simulink model "Models"  (R2016b)
settings: Solver=FixedStepAuto  StartTime=0.0  StopTime=100  FixedStep=0.05  RelTol=1e-3
model workspace (MAT data in the model file):
  index = Simulink.Signal
  index.DataType = 'double'
  index.Dimensions = 1
  index.DimensionsMode = 'Fixed'
  index.Complexity = 'real'
  index.SampleTime = -1
  index.SamplingMode = 'auto'
  index.InitialValue = '1'
values from neighbouring files (symbols this model uses):
  dpitch = 7.203    [Parameters.m]
  droll = 0.1094    [Parameters.m]
  dx = 2.86    [Parameters.m]
  dyaw = 0.26285    [Parameters.m]
  dz = 0    [Parameters.m]
  F = Fe(1:2,1:3)    [ControllerLQR.m]    (also in robustModel.m = -info.KFI(1:2,1:3))
  Ix = 0.06541    [Parameters.m]
  Iy = 1.08921    [Parameters.m]
  Iz = 1.10675    [Parameters.m]    (also in robustModel.m = Iz-0.22)
  l1 = 0.05    [Parameters.m]
  l2 = 0.05    [Parameters.m]
  m = 13    [Parameters.m]    (also in robustModel.m = m-2.6)
  refXdot = 1    [ControllerLQR.m]    (also in robustModel.m)
  refYaw = 1    [ControllerLQR.m]    (also in robustModel.m)
  Tpitch = 131.8316    [Parameters.m]
  Troll = 6.9736    [Parameters.m]
undefined symbols (not defined in the file or in its folder): DiscIntNeverNeededParam, F1, F2, Fi
settings Model: Creator=USUARIO  LastModifiedBy=aleja
settings DataIOCC: Refine=100

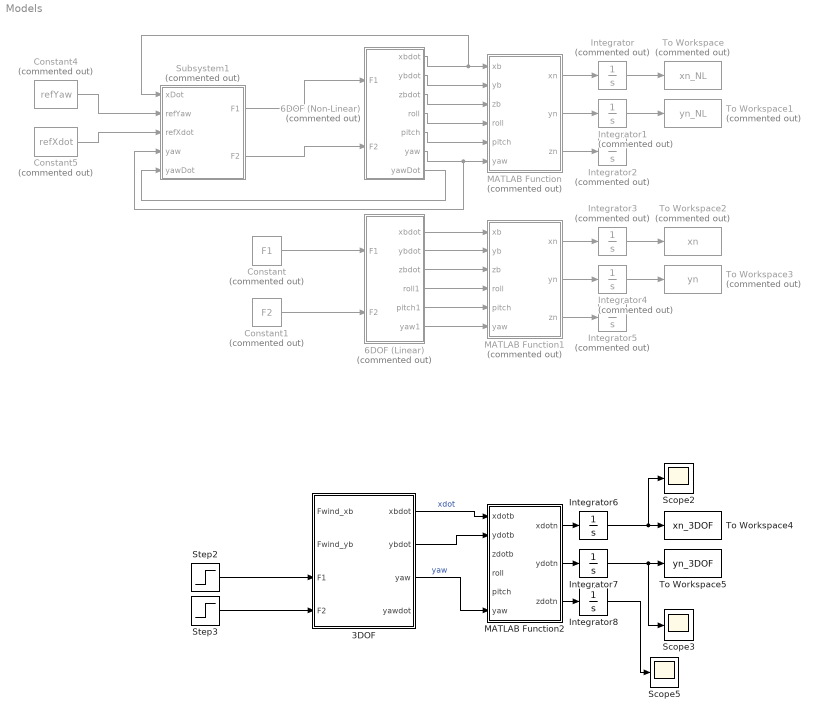
== system Models ==
  3DOF : Subsystem
  6DOF (Linear) : Subsystem  Commented=on
  6DOF (Non-Linear) : Subsystem  Commented=on
  Constant : Constant  Commented=on  Value=F1
  Constant1 : Constant  Commented=on  Value=F2
  Constant4 : Constant  Commented=on  Value=refYaw
  Constant5 : Constant  Commented=on  Value=refXdot
  Integrator{,1..5} (6 alike) : Integrator  Commented=on
  Integrator6 : Integrator
  Integrator7 : Integrator
  Integrator8 : Integrator
  MATLAB Function : MATLAB Function  Commented=on  TreatAsAtomicUnit=on
  MATLAB Function1 : MATLAB Function  Commented=on  TreatAsAtomicUnit=on
  MATLAB Function2 : MATLAB Function  TreatAsAtomicUnit=on
  Scope2 : Scope
  Scope3 : Scope
  Scope5 : Scope
  Step2 : Step  Time=10  After=14  SampleTime=0
  Step3 : Step  Time=10  After=14  SampleTime=0
  Subsystem1 : Subsystem  Commented=on
  To Workspace : ToWorkspace  Commented=on  VariableName=xn_NL  SaveFormat=Timeseries  SampleTime=-1
  To Workspace1 : ToWorkspace  Commented=on  VariableName=yn_NL  SaveFormat=Timeseries  SampleTime=-1
  To Workspace2 : ToWorkspace  Commented=on  VariableName=xn  SaveFormat=Timeseries  SampleTime=-1
  To Workspace3 : ToWorkspace  Commented=on  VariableName=yn  SaveFormat=Timeseries  SampleTime=-1
  To Workspace4 : ToWorkspace  VariableName=xn_3DOF  SaveFormat=Timeseries  SampleTime=-1
  To Workspace5 : ToWorkspace  VariableName=yn_3DOF  SaveFormat=Timeseries  SampleTime=-1
  wires:
  Constant/1 -> 6DOF (Linear)/1(F1)
  Constant1/1 -> 6DOF (Linear)/2(F2)
  MATLAB Function/1(xn) -> Integrator/1
  MATLAB Function/2(yn) -> Integrator1/1
  6DOF (Non-Linear)/6(yaw) -> Subsystem1/4(yaw), MATLAB Function/6(yaw)
  6DOF (Non-Linear)/5(pitch) -> MATLAB Function/5(pitch)
  6DOF (Non-Linear)/4(roll) -> MATLAB Function/4(roll)
  6DOF (Non-Linear)/3(zbdot) -> MATLAB Function/3(zb)
  6DOF (Non-Linear)/2(ybdot) -> MATLAB Function/2(yb)
  3DOF/1(xbdot) -> MATLAB Function2/1(xdotb)  "xdot"
  3DOF/2(ybdot) -> MATLAB Function2/2(ydotb)
  3DOF/3(yaw) -> MATLAB Function2/6(yaw)  "yaw"
  MATLAB Function1/1(xn) -> Integrator3/1
  MATLAB Function1/2(yn) -> Integrator4/1
  MATLAB Function/3(zn) -> Integrator2/1
  Integrator/1 -> To Workspace/1
  Integrator1/1 -> To Workspace1/1
  6DOF (Linear)/1(xbdot) -> MATLAB Function1/1(xb)
  6DOF (Linear)/2(ybdot) -> MATLAB Function1/2(yb)
  6DOF (Linear)/3(zbdot) -> MATLAB Function1/3(zb)
  6DOF (Linear)/4(roll1) -> MATLAB Function1/4(roll)
  6DOF (Linear)/5(pitch1) -> MATLAB Function1/5(pitch)
  6DOF (Linear)/6(yaw1) -> MATLAB Function1/6(yaw)
  Integrator3/1 -> To Workspace2/1
  Integrator4/1 -> To Workspace3/1
  MATLAB Function1/3(zn) -> Integrator5/1
  Integrator6/1 -> Scope2/1, To Workspace4/1
  Integrator7/1 -> Scope3/1, To Workspace5/1
  MATLAB Function2/3(zdotn) -> Integrator8/1
  6DOF (Non-Linear)/1(xbdot) -> Subsystem1/1(xDot), MATLAB Function/1(xb)
  Constant4/1 -> Subsystem1/2(refYaw)
  Constant5/1 -> Subsystem1/3(refXdot)
  Subsystem1/1(F1) -> 6DOF (Non-Linear)/1(F1)
  Subsystem1/2(F2) -> 6DOF (Non-Linear)/2(F2)
  6DOF (Non-Linear)/7(yawDot) -> Subsystem1/5(yawDot)
  MATLAB Function2/1(xdotn) -> Integrator6/1
  MATLAB Function2/2(ydotn) -> Integrator7/1
  Integrator8/1 -> Scope5/1
  Step2/1 -> 3DOF/3(F1)
  Step3/1 -> 3DOF/4(F2)

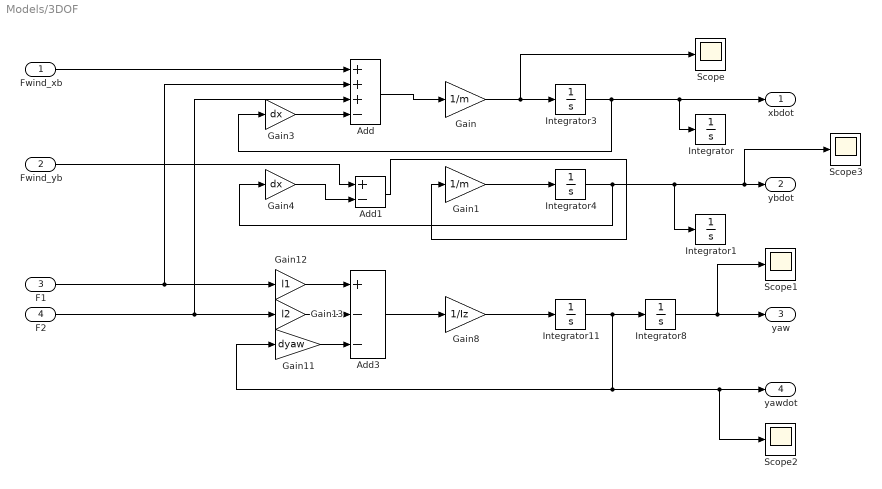
== system Models/3DOF ==
  Fwind_xb : Inport
  Fwind_yb : Inport  Port=2
  F1 : Inport  Port=3
  F2 : Inport  Port=4
  Add : Sum  Inputs=+++-
  Add1 : Sum  Inputs=+-
  Add3 : Sum  Inputs=+--
  Gain : Gain  Gain=1/m
  Gain1 : Gain  Gain=1/m
  Gain11 : Gain  Gain=dyaw
  Gain12 : Gain  Gain=l1
  Gain13 : Gain  Gain=l2
  Gain3 : Gain  Gain=dx
  Gain4 : Gain  Gain=dx
  Gain8 : Gain  Gain=1/Iz
  Integrator{,1,3..4,8,11} (6 alike) : Integrator
  Scope{,1..3} (4 alike) : Scope
  xbdot : Outport
  ybdot : Outport  Port=2
  yaw : Outport  Port=3
  yawdot : Outport  Port=4
  wires:
  Integrator11/1 -> Scope2/1, yawdot/1, Gain11/1, Integrator8/1
  Gain8/1 -> Integrator11/1
  Gain4/1 -> Add1/2
  Gain1/1 -> Integrator4/1
  Gain3/1 -> Add/4
  Add/1 -> Gain/1
  Gain/1 -> Scope/1, Integrator3/1
  Gain12/1 -> Add3/1
  Add3/1 -> Gain8/1
  Gain11/1 -> Add3/3
  Gain13/1 -> Add3/2
  Integrator3/1 -> Integrator/1, xbdot/1, Gain3/1
  Integrator4/1 -> Integrator1/1, Scope3/1, ybdot/1, Gain4/1
  Integrator8/1 -> Scope1/1, yaw/1
  F1/1 -> Add/2, Gain12/1
  F2/1 -> Add/3, Gain13/1
  Add1/1 -> Gain1/1
  Fwind_yb/1 -> Add1/1
  Fwind_xb/1 -> Add/1

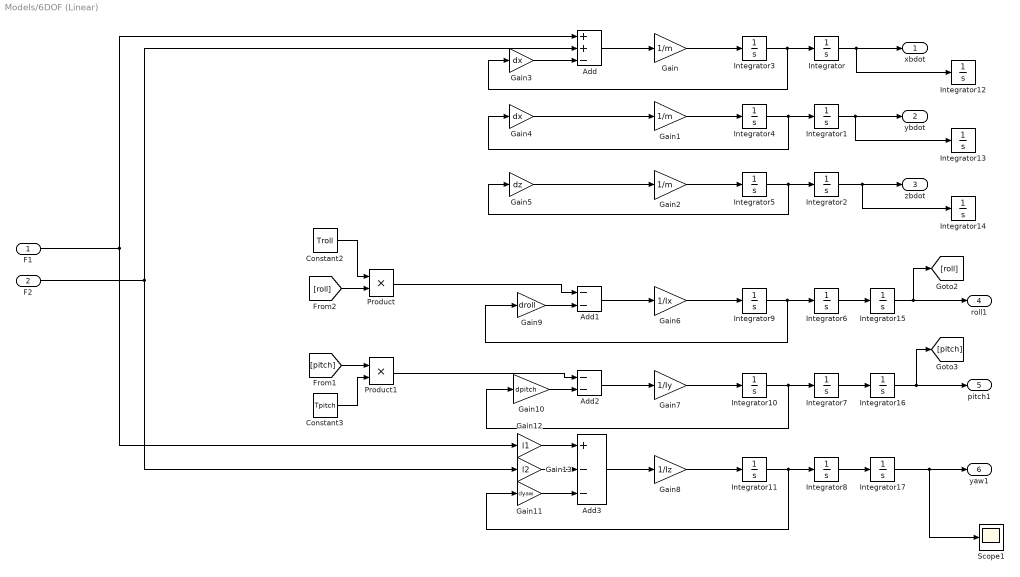
== system Models/6DOF (Linear) ==
  F1 : Inport
  F2 : Inport  Port=2
  Add : Sum  Inputs=++-
  Add1 : Sum  Inputs=--
  Add2 : Sum  Inputs=--
  Add3 : Sum  Inputs=+--
  Constant2 : Constant  Value=Troll
  Constant3 : Constant  Value=Tpitch
  Gain : Gain  Gain=1/m
  Gain1 : Gain  Gain=1/m
  Gain10 : Gain  Gain=dpitch
  Gain11 : Gain  Gain=dyaw
  Gain12 : Gain  Gain=l1
  Gain13 : Gain  Gain=l2
  Gain2 : Gain  Gain=1/m
  Gain3 : Gain  Gain=dx
  Gain4 : Gain  Gain=dx
  Gain5 : Gain  Gain=dz
  Gain6 : Gain  Gain=1/Ix
  Gain7 : Gain  Gain=1/Iy
  Gain8 : Gain  Gain=1/Iz
  Gain9 : Gain  Gain=droll
  Integrator{,1..17} (18 alike) : Integrator
  Product : Product
  Product1 : Product
  Scope1 : Scope
  xbdot : Outport
  ybdot : Outport  Port=2
  zbdot : Outport  Port=3
  roll1 : Outport  Port=4
  pitch1 : Outport  Port=5
  yaw1 : Outport  Port=6
  wires:
  Product/1 -> Add1/1
  Product1/1 -> Add2/1
  Gain9/1 -> Add1/2
  Gain13/1 -> Add3/2
  Gain11/1 -> Add3/3
  Add3/1 -> Gain8/1
  Constant2/1 -> Product/1
  Gain12/1 -> Add3/1
  Constant3/1 -> Product1/2
  Gain10/1 -> Add2/2
  Add2/1 -> Gain7/1
  Add1/1 -> Gain6/1
  Integrator6/1 -> Integrator15/1
  Integrator4/1 -> Integrator1/1, Gain4/1
  Gain/1 -> Integrator3/1
  Add/1 -> Gain/1
  F2/1 -> Add/2, Gain13/1
  Gain2/1 -> Integrator5/1
  Gain3/1 -> Add/3
  Gain1/1 -> Integrator4/1
  Gain5/1 -> Gain2/1
  Gain4/1 -> Gain1/1
  Integrator10/1 -> Integrator7/1, Gain10/1
  Gain8/1 -> Integrator11/1
  Integrator11/1 -> Integrator8/1, Gain11/1
  Gain7/1 -> Integrator10/1
  Gain6/1 -> Integrator9/1
  Integrator9/1 -> Integrator6/1, Gain9/1
  Integrator5/1 -> Integrator2/1, Gain5/1
  F1/1 -> Add/1, Gain12/1
  Integrator3/1 -> Integrator/1, Gain3/1
  [roll] -> Product/2
  [pitch] -> Product1/1
  Integrator2/1 -> Integrator14/1, zbdot/1
  Integrator17/1 -> Scope1/1, yaw1/1
  Integrator16/1 -> pitch1/1, [pitch]
  Integrator15/1 -> roll1/1, [roll]
  Integrator/1 -> Integrator12/1, xbdot/1
  Integrator1/1 -> Integrator13/1, ybdot/1
  Integrator7/1 -> Integrator16/1
  Integrator8/1 -> Integrator17/1

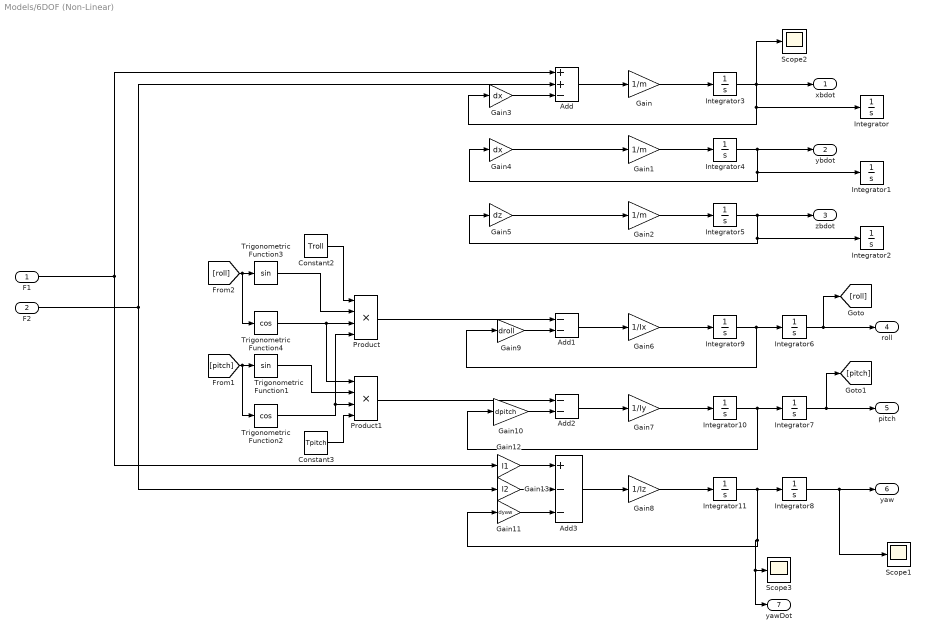
== system Models/6DOF (Non-Linear) ==
  F1 : Inport
  F2 : Inport  Port=2
  Add : Sum  Inputs=++-
  Add1 : Sum  Inputs=--
  Add2 : Sum  Inputs=--
  Add3 : Sum  Inputs=+--
  Constant2 : Constant  Value=Troll
  Constant3 : Constant  Value=Tpitch
  Gain : Gain  Gain=1/m
  Gain1 : Gain  Gain=1/m
  Gain10 : Gain  Gain=dpitch
  Gain11 : Gain  Gain=dyaw
  Gain12 : Gain  Gain=l1
  Gain13 : Gain  Gain=l2
  Gain2 : Gain  Gain=1/m
  Gain3 : Gain  Gain=dx
  Gain4 : Gain  Gain=dx
  Gain5 : Gain  Gain=dz
  Gain6 : Gain  Gain=1/Ix
  Gain7 : Gain  Gain=1/Iy
  Gain8 : Gain  Gain=1/Iz
  Gain9 : Gain  Gain=droll
  Integrator{,1..11} (12 alike) : Integrator
  Product : Product  Inputs=4
  Product1 : Product  Inputs=4
  Scope1 : Scope
  Scope2 : Scope
  Scope3 : Scope
  Trigonometric Function1 : Trigonometry
  Trigonometric Function2 : Trigonometry  Operator=cos
  Trigonometric Function3 : Trigonometry
  Trigonometric Function4 : Trigonometry  Operator=cos
  xbdot : Outport
  ybdot : Outport  Port=2
  zbdot : Outport  Port=3
  roll : Outport  Port=4
  pitch : Outport  Port=5
  yaw : Outport  Port=6
  yawDot : Outport  Port=7
  wires:
  F1/1 -> Gain12/1, Add/1
  Gain6/1 -> Integrator9/1
  Gain7/1 -> Integrator10/1
  Gain8/1 -> Integrator11/1
  Gain4/1 -> Gain1/1
  Gain5/1 -> Gain2/1
  Gain1/1 -> Integrator4/1
  Gain3/1 -> Add/3
  Gain2/1 -> Integrator5/1
  F2/1 -> Gain13/1, Add/2
  Add/1 -> Gain/1
  Gain/1 -> Integrator3/1
  Integrator9/1 -> Integrator6/1, Gain9/1
  Integrator10/1 -> Integrator7/1, Gain10/1
  Add1/1 -> Gain6/1
  Add2/1 -> Gain7/1
  Gain10/1 -> Add2/2
  Constant3/1 -> Product1/4
  Gain12/1 -> Add3/1
  Constant2/1 -> Product/1
  Add3/1 -> Gain8/1
  Gain11/1 -> Add3/3
  Gain13/1 -> Add3/2
  Gain9/1 -> Add1/2
  Product1/1 -> Add2/1
  Trigonometric Function4/1 -> Product1/1, Product/3
  Trigonometric Function1/1 -> Product1/2
  [pitch] -> Trigonometric Function2/1, Trigonometric Function1/1
  Trigonometric Function2/1 -> Product1/3, Product/4
  [roll] -> Trigonometric Function4/1, Trigonometric Function3/1
  Product/1 -> Add1/1
  Trigonometric Function3/1 -> Product/2
  Integrator5/1 -> zbdot/1, Integrator2/1, Gain5/1
  Integrator11/1 -> Integrator8/1, yawDot/1, Scope3/1, Gain11/1
  Integrator8/1 -> Scope1/1, yaw/1
  Integrator7/1 -> pitch/1, [pitch]
  Integrator6/1 -> roll/1, [roll]
  Integrator3/1 -> xbdot/1, Scope2/1, Integrator/1, Gain3/1
  Integrator4/1 -> ybdot/1, Integrator1/1, Gain4/1

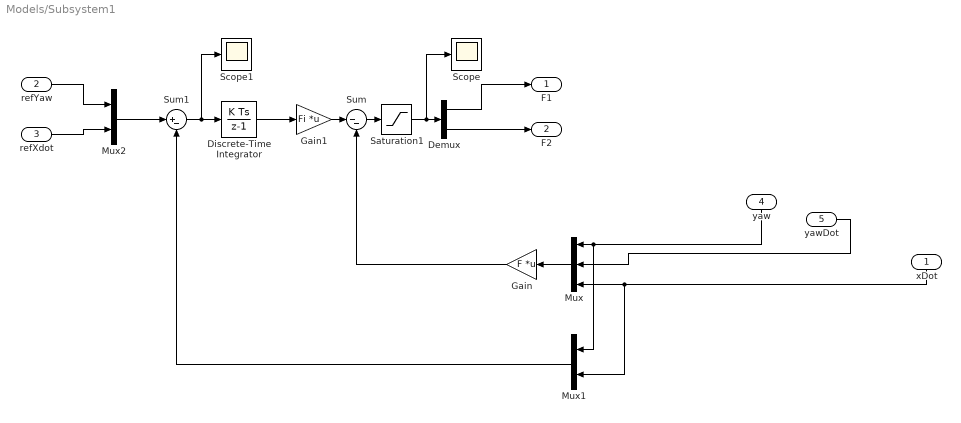
== system Models/Subsystem1 ==
  xDot : Inport
  refYaw : Inport  Port=2
  refXdot : Inport  Port=3
  yaw : Inport  Port=4
  yawDot : Inport  Port=5
  Demux : Demux  Outputs=2
  Discrete-Time Integrator : DiscreteIntegrator  InitialConditionSetting=State (most efficient)  SampleTime=-1  ICPrevOutput=DiscIntNeverNeededParam  ICPrevScaledInput=DiscIntNeverNeededParam
  Gain : Gain  Gain=F  Multiplication=Matrix(K*u)
  Gain1 : Gain  Gain=Fi  Multiplication=Matrix(K*u)
  Mux : Mux  Inputs=3
  Mux1 : Mux  Inputs=2
  Mux2 : Mux  Inputs=2
  Saturation1 : Saturate  UpperLimit=50  LowerLimit=-25
  Scope : Scope
  Scope1 : Scope
  Sum : Sum  Inputs=|--
  Sum1 : Sum  Inputs=|+-
  F1 : Outport
  F2 : Outport  Port=2
  wires:
  Gain1/1 -> Sum/1
  Saturation1/1 -> Scope/1, Demux/1
  xDot/1 -> Mux1/2, Mux/3
  yaw/1 -> Mux1/1, Mux/1
  Sum1/1 -> Scope1/1, Discrete-Time Integrator/1
  Demux/1 -> F1/1
  Demux/2 -> F2/1
  Discrete-Time Integrator/1 -> Gain1/1
  yawDot/1 -> Mux/2
  Sum/1 -> Saturation1/1
  Gain/1 -> Sum/2
  Mux/1 -> Gain/1
  refYaw/1 -> Mux2/1
  Mux2/1 -> Sum1/1
  Mux1/1 -> Sum1/2
  refXdot/1 -> Mux2/2

== matlab function Models/MATLAB Function1 ==
  data: xb input; xn output; yb input; zb input; roll input; pitch input; yaw input; yn output; zn output
function [xn,yn,zn] = fcn(xb,yb,zb,roll,pitch,yaw)
R=[cos(pitch)*cos(yaw) sin(roll)*sin(pitch)*cos(yaw)-cos(roll)*sin(yaw) ...
                          cos(roll)*sin(pitch)*cos(yaw)+sin(roll)*sin(yaw);
   cos(pitch)*sin(yaw) sin(roll)*sin(pitch)*sin(yaw)+cos(roll)*cos(yaw) ...
                          cos(roll)*sin(pitch)*sin(yaw)-sin(roll)*cos(yaw);
   -sin(pitch) sin(roll)*cos(pitch) cos(roll)*cos(pitch)];

n=R*[xb;yb;zb];

xn=n(1);
yn=n(2);
zn=n(3);
end

== matlab function Models/MATLAB Function ==
  data: xb input; xn output; yb input; zb input; roll input; pitch input; yaw input; yn output; zn output
function [xn,yn,zn] = fcn(xb,yb,zb,roll,pitch,yaw)
R=[cos(pitch)*cos(yaw) sin(roll)*sin(pitch)*cos(yaw)-cos(roll)*sin(yaw) ...
                          cos(roll)*sin(pitch)*cos(yaw)+sin(roll)*sin(yaw);
   cos(pitch)*sin(yaw) sin(roll)*sin(pitch)*sin(yaw)+cos(roll)*cos(yaw) ...
                          cos(roll)*sin(pitch)*sin(yaw)-sin(roll)*cos(yaw);
   -sin(pitch) sin(roll)*cos(pitch) cos(roll)*cos(pitch)];

n=R*[xb;yb;zb];

xn=n(1);
yn=n(2);
zn=n(3);
end

== matlab function Models/MATLAB Function2 ==
  data: xdotb input; xdotn output; ydotb input; zdotb input; roll input; pitch input; yaw input; ydotn output; zdotn output
function [xdotn,ydotn,zdotn] = fcn(xdotb,ydotb,zdotb,roll,pitch,yaw)
R=[cos(pitch)*cos(yaw) sin(roll)*sin(pitch)*cos(yaw)-cos(roll)*sin(yaw) ...
                          cos(roll)*sin(pitch)*cos(yaw)+sin(roll)*sin(yaw);
   cos(pitch)*sin(yaw) sin(roll)*sin(pitch)*sin(yaw)+cos(roll)*cos(yaw) ...
                          cos(roll)*sin(pitch)*sin(yaw)-sin(roll)*cos(yaw);
   -sin(pitch) sin(roll)*cos(pitch) cos(roll)*cos(pitch)];

n=R*[xdotb;ydotb;zdotb];

xdotn=n(1);
ydotn=n(2);
zdotn=n(3);
end
